simulink model "simulation"  (R2025b)
settings: Solver=VariableStepAuto  StartTime=0.0  StopTime=2e-5  RelTol=1e-3
libraries: commfilt2 x2, commdigbbndpm3 x1, commrandsrc3 x1
settings Model: Creator=Panos  LastModifiedBy=Panos

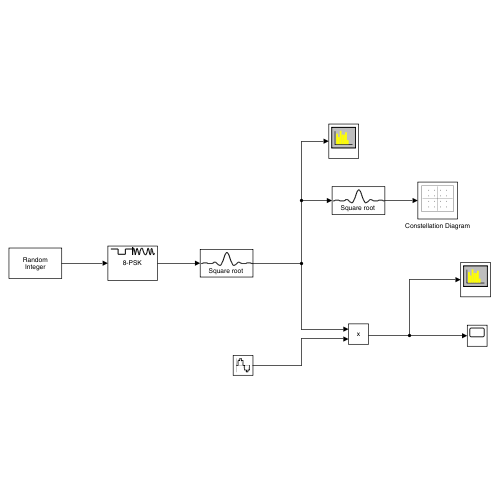
[thumbnail: Simulink's stored preview of the top-level diagram]
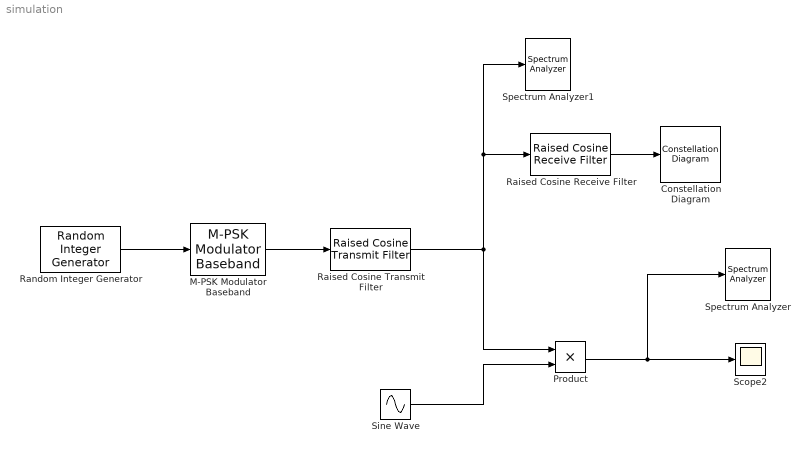
== system simulation ==
  Constellation Diagram : ConstellationDiagram  WindowPosition=[1.000000,49.000000,2048.000000,1081.000000,]  ScopeFrameLocation=window  SymbolsToDisplaySource=Property  SymbolsToDisplay=1000  ShowLegend=on
  M-PSK Modulator Baseband : commdigbbndpm3/M-PSK Modulator Baseband  M=8  InType=Integer  Enc=Gray  Mapping=[0:7]  Ph=pi/8  outDtype=double  outWordLen=16  outUDDataType=sfix(16)  outFracLenMode=Best precision  outFracLen=15  outDataTypeStr=double  outLastDataTypeStr=double
  Product : Product
  Raised Cosine Receive Filter : commfilt2/Raised Cosine Receive Filter  filtType=Square root  R=0.2  filtSpan=16  N=8  downFactor=8  downOffset=0  filterGain=1  InputProcessing=Columns as channels (frame based)  RateOptions=Allow multirate processing  framing=Mute  checkCoeff=off  variableName=rcRxFilt  currentFiltSpan=10  D=5  inputOffset=0  sampMode=Mute  saveAsFlag=0  rateMode=Downsampling  checkGain=Normalized  launchFVT=on  roundingMode=Floor  overflowMode=off  coeffDataTypeStr=Inherit: Same word length as input  coeffMin=[]  coeffMax=[]  coeffLastDataTypeStr=Inherit: Same word length as input  accumDataTypeStr=Inherit: Same as product output  accumLastDataTypeStr=Inherit: Same as product output  outputDataTypeStr=Inherit: Same as accumulator  outputMin=[]  outputMax=[]  outputLastDataTypeStr=Inherit: Same as accumulator
  Raised Cosine Transmit Filter : commfilt2/Raised Cosine Transmit Filter  filtType=Square root  R=0.2  filtSpan=16  N=8  filterGain=1  InputProcessing=Columns as channels (frame based)  RateOptions=Allow multirate processing  framing=Mute  checkCoeff=off  variableName=rcTxFilt  checkGain=Normalized  sampMode=Mute  saveAsFlag=0  currentFiltSpan=10  D=(10)/2  launchFVT=on  roundingMode=Floor  overflowMode=off  coeffDataTypeStr=Inherit: Same word length as input  coeffMin=[]  coeffMax=[]  coeffLastDataTypeStr=Inherit: Same word length as input  outputDataTypeStr=Inherit: Same as accumulator  outputMin=[]  outputMax=[]  outputLastDataTypeStr=Inherit: Same as accumulator
  Random Integer Generator : commrandsrc3/Random Integer Generator  SetSize=8  SeedSource=Auto  Seed=0  SampleTime=3e-9  SamplesPerFrame=1  OutputDataType=double  SimulateUsing=Interpreted execution
  Scope2 : Scope
      settings: ActiveDisplayYMinimum=-4.76197214608271  ActiveDisplayYMaximum=4.2001194669356758  DataLoggingVariableName=ScopeData2
  Sine Wave : Sin  Frequency=2*pi*30e9  SampleTime=1e-11
  Spectrum Analyzer : SpectrumAnalyzer  WindowPosition=[1.000000,49.000000,2048.000000,1081.000000,]  ScopeFrameLocation=window  PlotAsTwoSidedSpectrum=off  WindowInvariantSamplesPerUpdate=on  NumTapsPerBand=38  FilterSharpness=0.8  FrequencySpan=Span and center frequency  Span=10e9  CenterFrequency=30e9  StartFrequency=-50000000000  StopFrequency=50000000000  ReferenceLoad=50  YLimits=[-123.0659 5.8553]  ShowLegend=on  SelectedToolstripTab=spectrumAnalyzerToolstrip.estimationTab
  Spectrum Analyzer1 : SpectrumAnalyzer  WindowPosition=[1.000000,49.000000,2048.000000,1081.000000,]  ScopeFrameLocation=window  WindowInvariantSamplesPerUpdate=on  NumTapsPerBand=38  FilterSharpness=0.8  Span=2e9  CenterFrequency=30e9  StartFrequency=-50000000000  StopFrequency=50000000000  ReferenceLoad=50  YLimits=[-70.5423 -8.9333]  ShowLegend=on  SelectedToolstripTab=spectrumAnalyzerToolstrip.spectrumTab
  wires:
  Random Integer Generator/1 -> M-PSK Modulator Baseband/1
  Sine Wave/1 -> Product/2
  Product/1 -> Scope2/1, Spectrum Analyzer/1
  M-PSK Modulator Baseband/1 -> Raised Cosine Transmit Filter/1
  Raised Cosine Transmit Filter/1 -> Spectrum Analyzer1/1, Raised Cosine Receive Filter/1, Product/1
  Raised Cosine Receive Filter/1 -> Constellation Diagram/1
